simulink library "xrbsDSP_r3"  (Simulink 5.0)
undefined symbols (not defined in the file or in its folder): FIR1, Ft, mem
libraries: xbsIndex_r3 x329
(part 4 of 4)

== system xrbsDSP_r3/m-channel n-tap Transpose FIR Filter/MAD4 ==
  In1 : Inport
  In2 : Inport  Port=2
  AddSub : xbsIndex_r3/AddSub  mode=Addition  precision=User Defined  arith_type="Signed  (2's comp)"  n_bits=output_bitwidth  bin_pt=output_binpt  quantization=Truncate  overflow=Wrap  latency=channels  explicit_period=off  period=1  use_carryin=off  use_carryout=off  en=off  dbl_ovrd=off  show_param=off  use_core=on  pipeline=off  use_rpm=off  gen_core=on
      settings: xl_area=[32 64 0 64 0 0 0]
  Constant : xbsIndex_r3/Constant  const=coef  arith_type="Signed  (2's comp)"  n_bits=coef_bitwidth  bin_pt=coef_binpt  explicit_period=off  period=1  dbl_ovrd=off
  Mult : xbsIndex_r3/Mult  precision=Full  arith_type="Signed  (2's comp)"  n_bits=8  bin_pt=2  quantization=Truncate  overflow=Wrap  latency=2  explicit_period=off  period=1  en=off  dbl_ovrd=off  show_param=off  mult_type=Parallel  oversample=2  use_embedded=on  pipeline=on  use_rpm=off  placement_style=Rectangular Shape  gen_core=on
      settings: xl_area=[17 34 0 0 0 1 0]
  Out1 : Outport
  wires:
  In2/1 -> AddSub/2
  AddSub/1 -> Out1/1
  In1/1 -> Mult/1
  Constant/1 -> Mult/2
  Mult/1 -> AddSub/1

== system xrbsDSP_r3/m-channel n-tap Transpose FIR Filter/MAD5 ==
  In1 : Inport
  In2 : Inport  Port=2
  AddSub : xbsIndex_r3/AddSub  mode=Addition  precision=User Defined  arith_type="Signed  (2's comp)"  n_bits=output_bitwidth  bin_pt=output_binpt  quantization=Truncate  overflow=Wrap  latency=channels  explicit_period=off  period=1  use_carryin=off  use_carryout=off  en=off  dbl_ovrd=off  show_param=off  use_core=on  pipeline=off  use_rpm=off  gen_core=on
      settings: xl_area=[32 64 0 64 0 0 0]
  Constant : xbsIndex_r3/Constant  const=coef  arith_type="Signed  (2's comp)"  n_bits=coef_bitwidth  bin_pt=coef_binpt  explicit_period=off  period=1  dbl_ovrd=off
  Mult : xbsIndex_r3/Mult  precision=Full  arith_type="Signed  (2's comp)"  n_bits=8  bin_pt=2  quantization=Truncate  overflow=Wrap  latency=2  explicit_period=off  period=1  en=off  dbl_ovrd=off  show_param=off  mult_type=Parallel  oversample=2  use_embedded=on  pipeline=on  use_rpm=off  placement_style=Rectangular Shape  gen_core=on
      settings: xl_area=[17 34 0 0 0 1 0]
  Out1 : Outport
  wires:
  In2/1 -> AddSub/2
  AddSub/1 -> Out1/1
  In1/1 -> Mult/1
  Constant/1 -> Mult/2
  Mult/1 -> AddSub/1

== system xrbsDSP_r3/m-channel n-tap Transpose FIR Filter/MAD6 ==
  In1 : Inport
  In2 : Inport  Port=2
  AddSub : xbsIndex_r3/AddSub  mode=Addition  precision=User Defined  arith_type="Signed  (2's comp)"  n_bits=output_bitwidth  bin_pt=output_binpt  quantization=Truncate  overflow=Wrap  latency=channels  explicit_period=off  period=1  use_carryin=off  use_carryout=off  en=off  dbl_ovrd=off  show_param=off  use_core=on  pipeline=off  use_rpm=off  gen_core=on
      settings: xl_area=[32 64 0 64 0 0 0]
  Constant : xbsIndex_r3/Constant  const=coef  arith_type="Signed  (2's comp)"  n_bits=coef_bitwidth  bin_pt=coef_binpt  explicit_period=off  period=1  dbl_ovrd=off
  Mult : xbsIndex_r3/Mult  precision=Full  arith_type="Signed  (2's comp)"  n_bits=8  bin_pt=2  quantization=Truncate  overflow=Wrap  latency=2  explicit_period=off  period=1  en=off  dbl_ovrd=off  show_param=off  mult_type=Parallel  oversample=2  use_embedded=on  pipeline=on  use_rpm=off  placement_style=Rectangular Shape  gen_core=on
      settings: xl_area=[17 34 0 0 0 1 0]
  Out1 : Outport
  wires:
  In2/1 -> AddSub/2
  AddSub/1 -> Out1/1
  In1/1 -> Mult/1
  Constant/1 -> Mult/2
  Mult/1 -> AddSub/1

== system xrbsDSP_r3/m-channel n-tap Transpose FIR Filter/MAD7 ==
  In1 : Inport
  In2 : Inport  Port=2
  AddSub : xbsIndex_r3/AddSub  mode=Addition  precision=User Defined  arith_type="Signed  (2's comp)"  n_bits=output_bitwidth  bin_pt=output_binpt  quantization=Truncate  overflow=Wrap  latency=channels  explicit_period=off  period=1  use_carryin=off  use_carryout=off  en=off  dbl_ovrd=off  show_param=off  use_core=on  pipeline=off  use_rpm=off  gen_core=on
      settings: xl_area=[32 64 0 64 0 0 0]
  Constant : xbsIndex_r3/Constant  const=coef  arith_type="Signed  (2's comp)"  n_bits=coef_bitwidth  bin_pt=coef_binpt  explicit_period=off  period=1  dbl_ovrd=off
  Mult : xbsIndex_r3/Mult  precision=Full  arith_type="Signed  (2's comp)"  n_bits=8  bin_pt=2  quantization=Truncate  overflow=Wrap  latency=2  explicit_period=off  period=1  en=off  dbl_ovrd=off  show_param=off  mult_type=Parallel  oversample=2  use_embedded=on  pipeline=on  use_rpm=off  placement_style=Rectangular Shape  gen_core=on
      settings: xl_area=[17 34 0 0 0 1 0]
  Out1 : Outport
  wires:
  In2/1 -> AddSub/2
  AddSub/1 -> Out1/1
  In1/1 -> Mult/1
  Constant/1 -> Mult/2
  Mult/1 -> AddSub/1

== system xrbsDSP_r3/m-channel n-tap Transpose FIR Filter/MAD8 ==
  In1 : Inport
  In2 : Inport  Port=2
  AddSub : xbsIndex_r3/AddSub  mode=Addition  precision=User Defined  arith_type="Signed  (2's comp)"  n_bits=output_bitwidth  bin_pt=output_binpt  quantization=Truncate  overflow=Wrap  latency=channels  explicit_period=off  period=1  use_carryin=off  use_carryout=off  en=off  dbl_ovrd=off  show_param=off  use_core=on  pipeline=off  use_rpm=off  gen_core=on
      settings: xl_area=[32 64 0 64 0 0 0]
  Constant : xbsIndex_r3/Constant  const=coef  arith_type="Signed  (2's comp)"  n_bits=coef_bitwidth  bin_pt=coef_binpt  explicit_period=off  period=1  dbl_ovrd=off
  Mult : xbsIndex_r3/Mult  precision=Full  arith_type="Signed  (2's comp)"  n_bits=8  bin_pt=2  quantization=Truncate  overflow=Wrap  latency=2  explicit_period=off  period=1  en=off  dbl_ovrd=off  show_param=off  mult_type=Parallel  oversample=2  use_embedded=on  pipeline=on  use_rpm=off  placement_style=Rectangular Shape  gen_core=on
      settings: xl_area=[17 34 0 0 0 1 0]
  Out1 : Outport
  wires:
  In2/1 -> AddSub/2
  AddSub/1 -> Out1/1
  In1/1 -> Mult/1
  Constant/1 -> Mult/2
  Mult/1 -> AddSub/1

== system xrbsDSP_r3/m-channel n-tap Transpose FIR Filter/MAD9 ==
  In1 : Inport
  In2 : Inport  Port=2
  AddSub : xbsIndex_r3/AddSub  mode=Addition  precision=User Defined  arith_type="Signed  (2's comp)"  n_bits=output_bitwidth  bin_pt=output_binpt  quantization=Truncate  overflow=Wrap  latency=channels  explicit_period=off  period=1  use_carryin=off  use_carryout=off  en=off  dbl_ovrd=off  show_param=off  use_core=on  pipeline=off  use_rpm=off  gen_core=on
      settings: xl_area=[32 64 0 64 0 0 0]
  Constant : xbsIndex_r3/Constant  const=coef  arith_type="Signed  (2's comp)"  n_bits=coef_bitwidth  bin_pt=coef_binpt  explicit_period=off  period=1  dbl_ovrd=off
  Mult : xbsIndex_r3/Mult  precision=Full  arith_type="Signed  (2's comp)"  n_bits=8  bin_pt=2  quantization=Truncate  overflow=Wrap  latency=2  explicit_period=off  period=1  en=off  dbl_ovrd=off  show_param=off  mult_type=Parallel  oversample=2  use_embedded=on  pipeline=on  use_rpm=off  placement_style=Rectangular Shape  gen_core=on
      settings: xl_area=[17 34 0 0 0 1 0]
  Out1 : Outport
  wires:
  In2/1 -> AddSub/2
  AddSub/1 -> Out1/1
  In1/1 -> Mult/1
  Constant/1 -> Mult/2
  Mult/1 -> AddSub/1

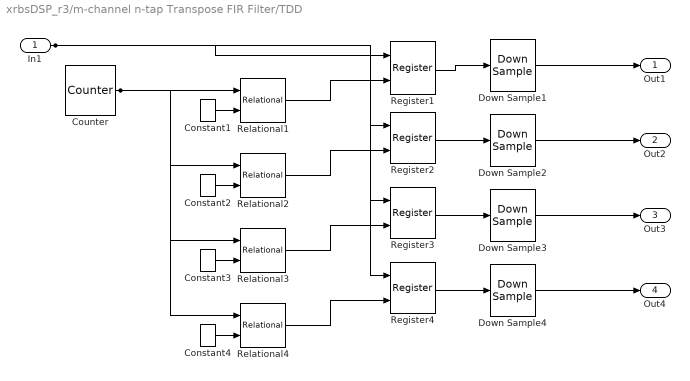
== system xrbsDSP_r3/m-channel n-tap Transpose FIR Filter/TDD ==
  In1 : Inport
  Constant1 : xbsIndex_r3/Constant  const=3  arith_type=Unsigned  n_bits=3  bin_pt=0  explicit_period=off  period=1  dbl_ovrd=off
  Constant2 : xbsIndex_r3/Constant  const=0  arith_type=Unsigned  n_bits=1  bin_pt=0  explicit_period=off  period=1  dbl_ovrd=off
  Constant3 : xbsIndex_r3/Constant  const=1  arith_type=Unsigned  n_bits=2  bin_pt=0  explicit_period=off  period=1  dbl_ovrd=off
  Constant4 : xbsIndex_r3/Constant  const=2  arith_type=Unsigned  n_bits=2  bin_pt=0  explicit_period=off  period=1  dbl_ovrd=off
  Counter : xbsIndex_r3/Counter  cnt_type=Count Limited  n_bits=2  bin_pt=0  arith_type=Unsigned  start_count=0  cnt_to=3  cnt_by_val=1  operation=Up  explicit_period=off  period=Ts/4  load_pin=off  rst=off  en=off  dbl_ovrd=off  show_param=off  use_rpm=on  gen_core=on
      settings: xl_area=[3 4 0 5 0 0 0]
  Down Sample{1..4} (4 alike) : xbsIndex_r3/Down Sample  sample_ratio=channels  sample_phase="Last Value of Frame  (most efficient)"  latency=1  en=off  dbl_ovrd=off  show_param=off
      settings: xl_area=[16 32 0 0 0 0 0]
  Register{1..4} (4 alike) : xbsIndex_r3/Register  init=0  reg_only_valid=off  explicit_period=off  period=1  rst=off  en=on  out_en=off  dbl_ovrd=off  show_param=off
      settings: xl_area=[16 32 0 0 0 0 0]
  Relational{1..4} (4 alike) : xbsIndex_r3/Relational  mode=a=b  latency=0  explicit_period=off  period=1  en=off  dbl_ovrd=off  show_param=off
      settings: xl_area=[1 0 0 2 0 0 0]
  Out1 : Outport
  Out2 : Outport  Port=2
  Out3 : Outport  Port=3
  Out4 : Outport  Port=4
  wires:
  Counter/1 -> Relational1/1, Relational2/1, Relational3/1, Relational4/1
  Constant1/1 -> Relational1/2
  Relational1/1 -> Register1/2
  In1/1 -> Register1/1, Register2/1, Register3/1, Register4/1
  Register1/1 -> Down Sample1/1
  Down Sample1/1 -> Out1/1
  Constant2/1 -> Relational2/2
  Relational2/1 -> Register2/2
  Register2/1 -> Down Sample2/1
  Down Sample2/1 -> Out2/1
  Constant3/1 -> Relational3/2
  Relational3/1 -> Register3/2
  Register3/1 -> Down Sample3/1
  Down Sample3/1 -> Out3/1
  Constant4/1 -> Relational4/2
  Relational4/1 -> Register4/2
  Register4/1 -> Down Sample4/1
  Down Sample4/1 -> Out4/1

== system xrbsDSP_r3/m-channel n-tap Transpose FIR Filter/TDM ==
  In1 : Inport
  In2 : Inport  Port=2
  In3 : Inport  Port=3
  In4 : Inport  Port=4
  Counter : xbsIndex_r3/Counter  cnt_type=Count Limited  n_bits=2  bin_pt=0  arith_type=Unsigned  start_count=0  cnt_to=3  cnt_by_val=1  operation=Up  explicit_period=off  period=Ts/4  load_pin=off  rst=off  en=off  dbl_ovrd=off  show_param=off  use_rpm=on  gen_core=off
      settings: xl_area=[0, 0, 0, 0, 0, 0, 0]
  Mux1 : xbsIndex_r3/Mux  inputs=4  precision=Full  arith_type="Signed  (2's comp)"  n_bits=8  bin_pt=2  quantization=Truncate  overflow=Wrap  latency=1  explicit_period=off  period=1  en=off  dbl_ovrd=off  show_param=off  mux_type=off  use_rpm=off  gen_core=off
      settings: xl_area=[0, 0, 0, 0, 0, 0, 0]
  Up Sample{1..4} (4 alike) : xbsIndex_r3/Up Sample  sample_ratio=channels  copy_samples=on  dbl_ovrd=off  show_param=off
      settings: xl_area=[0, 0, 0, 0, 0, 0, 0]
  Out1 : Outport
  wires:
  Counter/1 -> Mux1/1
  Mux1/1 -> Out1/1
  In1/1 -> Up Sample1/1
  Up Sample1/1 -> Mux1/2
  In2/1 -> Up Sample2/1
  Up Sample2/1 -> Mux1/3
  In3/1 -> Up Sample3/1
  Up Sample3/1 -> Mux1/4
  In4/1 -> Up Sample4/1
  Up Sample4/1 -> Mux1/5

== system xrbsDSP_r3/n-tap Dual Port Memory MAC FIR Filter/Address Control ==
  Coef Counter : xbsIndex_r3/Counter  Priority=5  cnt_type=Count Limited  n_bits=ceil(log2(2*length(coef)))  bin_pt=0  arith_type=Unsigned  start_count=length(coef)  cnt_to=2*length(coef)-1  cnt_by_val=1  operation=Up  explicit_period=off  period=Ts/length(coef)  load_pin=off  rst=off  en=off  dbl_ovrd=off  use_rpm=on  gen_core=on
      settings: xl_area=[0, 0, 0, 0, 0, 0, 0]
  Data  Counter : xbsIndex_r3/Counter  Priority=5  cnt_type=Count Limited  n_bits=ceil(log2(2*length(coef)))  bin_pt=0  arith_type=Unsigned  start_count=0  cnt_to=length(coef)-1  cnt_by_val=1  operation=Up  explicit_period=off  period=Ft/length(coef)  load_pin=off  rst=off  en=on  dbl_ovrd=off  use_rpm=on  gen_core=on
      settings: xl_area=[0, 0, 0, 0, 0, 0, 0]
  Delay1 : xbsIndex_r3/Delay  latency=1  reg_retiming=off  explicit_period=off  period=1  en=off  accept_only_valid=off  init_zero=on  dbl_ovrd=off
      settings: xl_area=[0, 0, 0, 0, 0, 0, 0]
  Inverter : xbsIndex_r3/Inverter  latency=0  explicit_period=off  period=1  en=off  dbl_ovrd=off
      settings: xl_area=[0, 0, 0, 0, 0, 0, 0]
  Relational1 : xbsIndex_r3/Relational  mode=a=b  latency=0  explicit_period=on  period=-1  en=off  dbl_ovrd=off
      settings: xl_area=[0, 0, 0, 0, 0, 0, 0]
  Zero1 : xbsIndex_r3/Constant  Priority=5  const=2*length(coef)-1  arith_type=Unsigned  n_bits=ceil(log2(2*length(coef)-1))  bin_pt=0  explicit_period=off  period=Ft/length(coef)  dbl_ovrd=off
  data_addr : Outport
  we : Outport  Port=2
  coef_addr : Outport  Port=3
  rst : Outport  Port=4
  wires:
  Inverter/1 -> Data  Counter/1
  Delay1/1 -> rst/1, we/1
  Relational1/1 -> Delay1/1, Inverter/1
  Zero1/1 -> Relational1/2
  Data  Counter/1 -> data_addr/1
  Coef Counter/1 -> Relational1/1, coef_addr/1

== system xrbsDSP_r3/n-tap Dual Port Memory MAC FIR Filter/Dual Port RAM ==
  note: The 'Unpad' subsystem removes the padded
      | bits when necessary,
  note: The 'Pad' and 'Unpad' subsystems concatenate zeros
      | on to the data stream if the coefficient bit width is
      | larger than the data width. They must be the same
      | size to be stored in block ram.
  din : Inport
  data_addr : Inport  Port=2
  we : Inport  Port=3
  coef_addr : Inport  Port=4
  Convert : xbsIndex_r3/Convert  arith_type="Signed  (2's comp)"  n_bits=coef_bit_width  bin_pt=coef_bin_pt  quantization=Truncate  overflow=Wrap  latency=0  explicit_period=off  period=1  dbl_ovrd=off  inserted_by_tool=off
      settings: xl_area=[0 0 0 0 0 0 0]
  Dual Port RAM : xbsIndex_r3/Dual Port RAM  depth=length(coef)*2  initVector=[zeros(1, length(coef)) coef(:)']  write_mode_A=Read After Write  write_mode_B=Read After Write  latency=1  distributed_mem=off  mem_collision=off  init_zero=on  explicit_period=off  period=1  dbl_ovrd=off  rst_a=off  init_a=0  rst_b=off  init_b=0  use_rpm=off  gen_core=on
      settings: xl_area=[0, 0, 0, 0, 0, 0, 0]
  Pad : Subsystem
  Unpad : Subsystem
  Up Sample : xbsIndex_r3/Up Sample  sample_ratio=length(coef)  copy_samples=on  dbl_ovrd=off
      settings: xl_area=[0, 0, 0, 0, 0, 0, 0]
  Zero : xbsIndex_r3/Constant  Priority=5  const=0  arith_type="Signed  (2's comp)"  n_bits=coef_bit_width + coef_pad_bits  bin_pt=coef_bin_pt  explicit_period=off  period=Ft/length(coef)  dbl_ovrd=off
  Zero1 : xbsIndex_r3/Constant  Priority=5  const=0  arith_type=Boolean  n_bits=1  bin_pt=0  explicit_period=off  period=Ft/length(coef)  dbl_ovrd=off
  dout_a : Outport
  dout_b : Outport  Port=2
  wires:
  Convert/1 -> dout_b/1
  Up Sample/1 -> Pad/1(din)
  Pad/1(dout) -> Dual Port RAM/2
  coef_addr/1 -> Dual Port RAM/4
  we/1 -> Dual Port RAM/3
  Unpad/1(dout) -> dout_a/1
  data_addr/1 -> Dual Port RAM/1
  din/1 -> Up Sample/1
  Dual Port RAM/1 -> Unpad/1(din)
  Zero1/1 -> Dual Port RAM/6
  Zero/1 -> Dual Port RAM/5
  Dual Port RAM/2 -> Convert/1

== system xrbsDSP_r3/n-tap MAC FIR Filter/MAC Engine ==
  note: The Multiplier block is implemented using Virtex-II  dedicated multipliers.
      | Enabling the 'Pipeline to Greatest Extent Possible' mask configuration
      | parameter ensures the internal pipeline stages of the dedicated
      | multipliers are used.
  note: This subsystem implements a multiply-accumulate engine.
  note: Upon reset, the accumulator reinitializes to its current input value
      | rather than zero, which allows the MAC engine to stream data without
      | stalling for one sample period.
  note: The precision required for the multiplier and the accumulator is a
      | function of the filter taps (coefficients) and the number of taps. Since
      | these are fixed at design time, it is possible to tailor the hardware resources
      | to the filter specification.  The multiplier need only have enough  bits to
      | compute the product of the largest magnitude coefficient and the largest
      | magnitude data input value.   That is,
      |
      |         mult_nbits = ceil(log2(max(abs(coef*2^coef_binpt))))+input_nbits + 1;
      |         mult_binpt = input_binpt+coef_binpt;
      |
      | Similarly, the accumulator need only have sufficient precision to accumulate
      | maximal input against the filter taps.
      |
      |         acc_nbits = ceil(log2(sum(abs(coef*2^coef_binpt)))) + input_nbits + 1;
      |         acc_binpt = mult_binpt;
      |
      | These variables are passed to the blocks as mask parameters.
  a : Inport
  b : Inport  Port=2
  rst : Inport  Port=3
  Accumulator : xbsIndex_r3/Accumulator  n_bits=ceil(log2(max(1,sum(abs(coef*2^coef_bin_pt)))))+smpl_n_bits + 1  overflow=Wrap  operation=Add  scale=1  explicit_period=off  period=1  rst=on  hasbypass=on  en=off  dbl_ovrd=off  show_param=off  gen_core=on  use_rpm=off
      settings: xl_area=[0, 0, 0, 0, 0, 0, 0]
  Mult : xbsIndex_r3/Mult  precision=User Defined  arith_type="Signed  (2's comp)"  n_bits=max(ceil(log2(max(1,max(abs(coef*2^coef_bin_pt)))))+smpl_n_bits + 1,smpl_bin_pt+coef_bin_pt)  bin_pt=smpl_bin_pt+coef_bin_pt  quantization=Truncate  overflow=Wrap  latency=2  explicit_period=off  period=1  en=off  dbl_ovrd=off  show_param=off  mult_type=Parallel  oversample=2  use_embedded=on  pipeline=on  use_rpm=on  placement_style=Rectangular Shape  gen_core=on
      settings: xl_area=[0, 0, 0, 0, 0, 0, 0]
  q : Outport
  wires:
  rst/1 -> Accumulator/2
  b/1 -> Mult/2
  Accumulator/1 -> q/1
  a/1 -> Mult/1
  Mult/1 -> Accumulator/1

== system xrbsDSP_r3/Dual Port Memory Interpolation MAC FIR Filter/Dual Port RAM/pad ==
  din : Inport
  Convert : xbsIndex_r3/Convert  arith_type="Signed  (2's comp)"  n_bits=bit_width + data_pad_bits  bin_pt=bin_pt  quantization=Truncate  overflow=Wrap  latency=0  explicit_period=off  period=1  dbl_ovrd=off  inserted_by_tool=off
      settings: xl_area=[0 0 0 0 0 0 0]
  Reinterpret : xbsIndex_r3/Reinterpret  force_arith_type=on  arith_type="Signed  (2's comp)"  force_bin_pt=on  bin_pt=coef_bin_pt  force_valid=on
  dout : Outport
  wires:
  Reinterpret/1 -> dout/1
  din/1 -> Convert/1
  Convert/1 -> Reinterpret/1

== system xrbsDSP_r3/Dual Port Memory Interpolation MAC FIR Filter/Dual Port RAM/unpad ==
  din : Inport
  Reinterpret : xbsIndex_r3/Reinterpret  force_arith_type=on  arith_type="Signed  (2's comp)"  force_bin_pt=on  bin_pt=bin_pt  force_valid=off
  Slice : xbsIndex_r3/Slice  mode=Lower Bit Location + Width  nbits=bit_width  bit1=0  base1=MSB of Input  bit0=0  base0=LSB of Input  boolean_output=off  explicit_period=off  period=1  dbl_ovrd=off
  dout : Outport
  wires:
  Reinterpret/1 -> dout/1
  din/1 -> Slice/1
  Slice/1 -> Reinterpret/1

== system xrbsDSP_r3/n-tap Dual Port Memory MAC FIR Filter/Dual Port RAM/Pad ==
  din : Inport
  Convert : xbsIndex_r3/Convert  arith_type="Signed  (2's comp)"  n_bits=bit_width + data_pad_bits  bin_pt=bin_pt  quantization=Truncate  overflow=Wrap  latency=0  explicit_period=off  period=1  dbl_ovrd=off  inserted_by_tool=off
      settings: xl_area=[0 0 0 0 0 0 0]
  Reinterpret : xbsIndex_r3/Reinterpret  force_arith_type=on  arith_type="Signed  (2's comp)"  force_bin_pt=on  bin_pt=coef_bin_pt  force_valid=on
  dout : Outport
  wires:
  Reinterpret/1 -> dout/1
  din/1 -> Convert/1
  Convert/1 -> Reinterpret/1

== system xrbsDSP_r3/n-tap Dual Port Memory MAC FIR Filter/Dual Port RAM/Unpad ==
  din : Inport
  Reinterpret : xbsIndex_r3/Reinterpret  force_arith_type=on  arith_type="Signed  (2's comp)"  force_bin_pt=on  bin_pt=bin_pt  force_valid=off
  Slice : xbsIndex_r3/Slice  mode=Lower Bit Location + Width  nbits=bit_width  bit1=0  base1=MSB of Input  bit0=0  base0=LSB of Input  boolean_output=off  explicit_period=off  period=1  dbl_ovrd=off
  dout : Outport
  wires:
  Reinterpret/1 -> dout/1
  din/1 -> Slice/1
  Slice/1 -> Reinterpret/1
